simulink model "kcm_cosim"  (Simulink 7.8)
settings: Solver=FixedStepDiscrete  SolverMode=SingleTasking  StartTime=0.0  StopTime=1e-1  RelTol=1e-3
undefined symbols (not defined in the file or in its folder): pipeline_prec
libraries: modelsimlib x5
Description:
  | Associated .vhd file: kcm_simulink_cosim_tb.vhd
settings Model: Creator=obmun  LastModifiedBy=obmun
settings OptimizationCC: InitFltsAndDblsToZero=on
settings DebuggingCC: SaveWithParameterizedLinksMsg=none  SignalResolutionControl=TryResolveAllWithWarning  MultiTaskDSMMsg=warning  MultiTaskCondExecSysMsg=none  FcnCallInpInsideContextMsg=Use local settings  StrictBusMsg=Warning
settings SFSimCC: SimParseCustomCode=off
settings RTWCC: IncludeERTFirstTime=on
settings GRTTargetCC: TargetFcnLib=ansi_tfl_tmw.mat

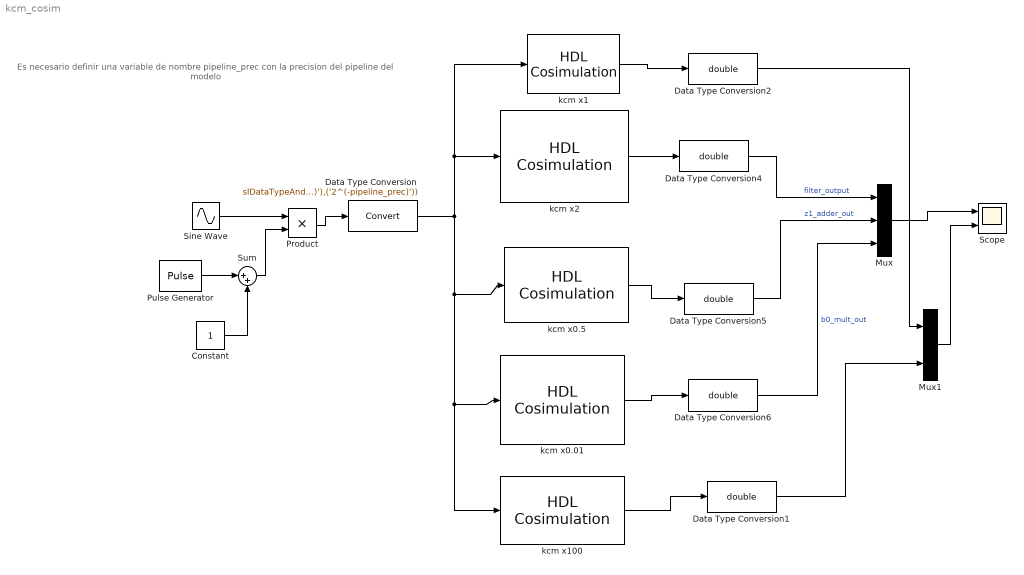
== system kcm_cosim ==
  note: Es necesario definir una variable de nombre pipeline_prec
      | con la precision del pipeline del modelo
  Constant : Constant
  Data Type Conversion : DataTypeConversion  OutDataTypeStr=slDataTypeAndScale(('sfix(16)'),('2^(-pipeline_prec)'))  RndMeth=Nearest  SampleTime=1e-4  SaturateOnIntegerOverflow=on
  Data Type Conversion{1..2,4..6} (5 alike) : DataTypeConversion  OutDataTypeStr=double
  Mux : Mux  Inputs=3
  Mux1 : Mux  Inputs=2
  Product : Product  RndMeth=Zero
  Pulse Generator : DiscretePulseGenerator  PulseType=Time based  Amplitude=4  Period=2/50  PulseWidth=50
  Scope : Scope  NumInputPorts=2
      settings: TimeRange=0.003858569876969357  YMin=-0.003846455865942407~-5  YMax=-0.003630890666446729~5  MaxDataPoints=500000
  Sine Wave : Sin  Frequency=2*pi*50
  Sum : Sum  Inputs=|++
  kcm x0.01 : modelsimlib/HDL Cosimulation  PortPaths=/kcm_cosim_tb/kcm_001_i/i;/kcm_cosim_tb/kcm_001_i/o  PortModes=[1 2 ]  PortTimes=[1,1e-4]  PortSigns=[-1 1 ]  PortFracLengths=[0,pipeline_prec]  CommLocal=on  CommSharedMemory=off  CommPortNumber=4449  CommShowInfo=on  ClockModes=[]  ClockTimes=[]  TclPreSimCommand="echo \"Running Simulink Cosimulation block.\""  TclPostSimCommand="echo \"done\""  TimingMode=s  TimingScaleFactor=1  idxCellArray={'UNUSED_VAR'}  CosimBypass=Full Simulation  AllowDirectFeedthrough=off  ProductName=EDA Simulator Link MQ  RunAutoTimescale=off  HdlClocks=0
  kcm x0.5 : modelsimlib/HDL Cosimulation  PortPaths=/kcm_cosim_tb/kcm_05_i/i;/kcm_cosim_tb/kcm_05_i/o  PortModes=[1 2 ]  PortTimes=[1,1e-4]  PortSigns=[-1 1 ]  PortFracLengths=[0,pipeline_prec]  CommLocal=on  CommSharedMemory=off  CommPortNumber=4449  CommShowInfo=on  ClockModes=[]  ClockTimes=[]  TclPreSimCommand="echo \"Running Simulink Cosimulation block.\""  TclPostSimCommand="echo \"done\""  TimingMode=s  TimingScaleFactor=1  idxCellArray={'UNUSED_VAR'}  CosimBypass=Full Simulation  AllowDirectFeedthrough=off  ProductName=EDA Simulator Link MQ  RunAutoTimescale=off  HdlClocks=0
  kcm x1 : modelsimlib/HDL Cosimulation  PortPaths=/kcm_cosim_tb/kcm_m233_i/i;/kcm_cosim_tb/kcm_m233_i/o  PortModes=[1 2 ]  PortTimes=[1,1e-4]  PortSigns=[-1 1 ]  PortFracLengths=[0,pipeline_prec]  CommLocal=on  CommSharedMemory=off  CommPortNumber=4449  CommShowInfo=on  ClockModes=[]  ClockTimes=[]  TclPreSimCommand="echo \"Running Simulink Cosimulation block.\""  TclPostSimCommand="echo \"done\""  TimingMode=s  TimingScaleFactor=1  idxCellArray={'UNUSED_VAR'}  CosimBypass=Full Simulation  AllowDirectFeedthrough=off  ProductName=EDA Simulator Link MQ  RunAutoTimescale=off  HdlClocks=0
  kcm x100 : modelsimlib/HDL Cosimulation  PortPaths=/kcm_cosim_tb/kcm_100_i/i;/kcm_cosim_tb/kcm_100_i/o  PortModes=[1 2 ]  PortTimes=[1,1e-4]  PortSigns=[-1 1 ]  PortFracLengths=[0,pipeline_prec]  CommLocal=on  CommSharedMemory=off  CommPortNumber=4449  CommShowInfo=on  ClockModes=[]  ClockTimes=[]  TclPreSimCommand="echo \"Running Simulink Cosimulation block.\""  TclPostSimCommand="echo \"done\""  TimingMode=s  TimingScaleFactor=1  idxCellArray={'UNUSED_VAR'}  CosimBypass=Full Simulation  AllowDirectFeedthrough=off  ProductName=EDA Simulator Link MQ  RunAutoTimescale=off  HdlClocks=0
  kcm x2 : modelsimlib/HDL Cosimulation  PortPaths=/kcm_cosim_tb/kcm_2_i/i;/kcm_cosim_tb/kcm_2_i/o  PortModes=[1 2 ]  PortTimes=[1,1e-4]  PortSigns=[-1 1 ]  PortFracLengths=[0,pipeline_prec]  CommLocal=on  CommSharedMemory=off  CommPortNumber=4449  CommShowInfo=on  ClockModes=[]  ClockTimes=[]  TclPreSimCommand="echo \"Running Simulink Cosimulation block.\""  TclPostSimCommand="echo \"done\""  TimingMode=s  TimingScaleFactor=1  idxCellArray={'UNUSED_VAR'}  CosimBypass=Full Simulation  AllowDirectFeedthrough=off  ProductName=EDA Simulator Link MQ  RunAutoTimescale=off  HdlClocks=0
  wires:
  Data Type Conversion/1 -> kcm x0.5/1, kcm x0.01/1, kcm x100/1, kcm x2/1, kcm x1/1
  kcm x2/1 -> Data Type Conversion4/1
  kcm x0.5/1 -> Data Type Conversion5/1
  kcm x0.01/1 -> Data Type Conversion6/1
  kcm x100/1 -> Data Type Conversion1/1
  Data Type Conversion4/1 -> Mux/1  "filter_output"
  Data Type Conversion5/1 -> Mux/2  "z1_adder_out"
  Data Type Conversion6/1 -> Mux/3  "b0_mult_out"
  Mux/1 -> Scope/1
  Pulse Generator/1 -> Sum/1
  Constant/1 -> Sum/2
  Sine Wave/1 -> Product/1
  Product/1 -> Data Type Conversion/1
  Sum/1 -> Product/2
  Mux1/1 -> Scope/2
  Data Type Conversion1/1 -> Mux1/2
  kcm x1/1 -> Data Type Conversion2/1
  Data Type Conversion2/1 -> Mux1/1
